simulink model "gm_uz_mpc_3ph"  (R2021a)
settings: Solver=FixedStepDiscrete  StartTime=0.0  StopTime=2000*t_ADC  RelTol=1e-3
undefined symbols (not defined in the file or in its folder): IB, id_ref, iq_ref, lambda_d, lambda_q, lambda_u, Ld_over_LB, Lq_over_LB, n_rpm, omegaB, p, psi_pm_over_psiB, Rs_over_ZB, t_ADC, t_clock, Ts_times_ZB_over_Ld, Ts_times_ZB_over_Lq, v_dc, VB
libraries: nesl_utility x19, simulink x18, fl_lib x15, ee_lib x7, hdlsllib x2, spsAlphaBetaZerotodq0Lib x1
(part 3 of 3)

== system gm_uz_mpc_3ph/inverter_machine/DC_link ==
  Capacitor : fl_lib/Electrical/Electrical Elements/Capacitor  c=C_dc_link uF  r=1e-6 Ohm  g=0 1/Ohm  i_specify=off  i_priority=None  i=0 A  i_nominal_specify=off  i_nominal_unit=A  i_nominal_value=1  v_specify=off  v_priority=None  v=0 V  v_nominal_specify=off  v_nominal_unit=V  v_nominal_value=1  vc_specify=off  vc_priority=High  vc=0 V  vc_nominal_specify=off  vc_nominal_unit=V  vc_nominal_value=1
  PS-Simulink Converter : nesl_utility/PS-Simulink Converter  PhysicalDomain=network_engine_domain  SubClassName=ps_output  LeftPortType=input  RightPortType=output  PseudoPeriodic=off  Frequencies=[]  Unit=1  AffineConversion=off
      settings: SourceProductBaseCode=PW,SS
  Voltage Sensor : fl_lib/Electrical/Electrical Sensors/Voltage Sensor
  U_dc_link+_in : PMIOPort  Side=Left
  U_dc_link-_in : PMIOPort  Port=2  Side=Left
  U_dc_link+_out : PMIOPort  Port=3  Side=Right
  U_dc_link-_out : PMIOPort  Port=4  Side=Right
  u_dc_link_measured : Outport  VectorParamsAs1DForOutWhenUnconnected=off
  wires:
  PS-Simulink Converter/1 -> u_dc_link_measured/1
  connections:
  Voltage Sensor/RConn1 -- PS-Simulink Converter/LConn1
  Capacitor/RConn1 -- U_dc_link-_out/RConn1 -- Voltage Sensor/RConn2 -- U_dc_link-_in/RConn1
  Capacitor/LConn1 -- U_dc_link+_out/RConn1 -- Voltage Sensor/LConn1 -- U_dc_link+_in/RConn1

== system gm_uz_mpc_3ph/inverter_machine/Power_Source ==
  Controlled Voltage Source : fl_lib/Electrical/Electrical Sources/Controlled Voltage Source
  + : PMIOPort  Side=Right
  - : PMIOPort  Port=2  Side=Right
  ref_voltage : PMIOPort  Port=3  Side=Left
  connections:
  Controlled Voltage Source/RConn1 -- ref_voltage/RConn1
  Controlled Voltage Source/RConn2 -- -/RConn1
  Controlled Voltage Source/LConn1 -- +/RConn1

== matlab function gm_uz_mpc_3ph/pu_voltages_vsd/finite_control_set ==
  settings: fimath=fimath('RoundingMethod', 'Floor','OverflowAction', 'Wrap','ProductMode', 'FullPrecision', 'SumMode', 'FullPrecision')
  data: v_DC_pu input; sin_angle input; pu_ud output; pu_uq output; cos_angle input; index input
function [pu_ud,pu_uq] = voltage_space_vectors(v_DC_pu, sin_angle, cos_angle, index)

fm = fimath();
v_DC_pu = fi(v_DC_pu,1,18,15,fm);
sin_angle = fi(sin_angle,1,27,20,fm);
cos_angle = fi(cos_angle,1,27,20,fm);

% u_d-voltages lookup factors alpha/beta
vd_pu = fi([0,0;
    0.666666666666667,0;
    -0.333333333333334,0.577350269189626;
    0.333333333333333,0.577350269189626;
    -0.333333333333333,-0.577350269189626;
    0.333333333333334,-0.577350269189626;
    -0.666666666666667,0;
    0,0],1,18,15);

% u_q-voltages lookup factors alpha/beta
vq_pu = fi([0,0;
    0.666666666666667,0;
    -0.333333333333334,0.577350269189626;
    0.333333333333333,0.577350269189626;
    -0.333333333333333,-0.577350269189626;
    0.333333333333334,-0.577350269189626;
    -0.666666666666667,0;
    0,0],1,18,15);

pu_ud = fi(v_DC_pu * (vd_pu(index,1) * cos_angle + vd_pu(index,2) * sin_angle),1,27,24);
pu_uq = fi(v_DC_pu * (vq_pu(index,1) * -sin_angle + vq_pu(index,2) * cos_angle),1,27,24);

== matlab function gm_uz_mpc_3ph/uz_clarke/clarke ==
  settings: fimath=fimath('RoundingMethod', 'Floor','OverflowAction', 'Wrap','ProductMode', 'FullPrecision', 'SumMode', 'FullPrecision')
  data: a1 input; alpha output; b1 input; c1 input; beta output; zero output
function [alpha,beta,zero] = fcn(a1,b1,c1)


A = [fi(0,1,18,11) fi(0,1,18,11) fi(0,1,18,11)]';

A =    2/3*[1    -0.5        -0.5       ;
           0    sqrt(3)/2   -sqrt(3)/2  ;
           0.5    0.5        0.5] * [a1 b1 c1 ]';

alpha = fi(A(1),1,18,11);
beta = fi(A(2),1,18,11);
zero = fi(A(3),1,18,11);

== matlab function gm_uz_mpc_3ph/cost_opt/MATLAB Function ==
  settings: fimath=fimath('RoundingMethod', 'Floor','OverflowAction', 'Wrap','ProductMode', 'FullPrecision', 'SumMode', 'FullPrecision')
  data: in input; G_next output; index input; last_optim_index input; G_prev output
function [G_next,G_prev] = get_switch_positions(in,index,last_optim_index)
%#codegen
G_next = in(index,[1 3 5]);
G_prev = in(last_optim_index,[1 3 5]);

== matlab function gm_uz_mpc_3ph/cost_opt/iterativesearch ==
  settings: fimath=fimath('RoundingMethod', 'Floor','OverflowAction', 'Wrap','ProductMode', 'FullPrecision', 'SumMode', 'FullPrecision')
  data: index input; opt_idx output; cost input; min_costs output; opt_done output
function [opt_idx,min_costs,opt_done] = fcn(index, cost)
%#codegen

persistent cost_old
if isempty(cost_old)
    cost_old = fi(4.98,0,27,24);
end

persistent index_old
if isempty(index_old)
    index_old = uint32(1);
end

persistent opt_idx_old
if isempty(opt_idx_old)
    opt_idx_old = uint32(1);
end

opt_done = false;

if (index ~= index_old)
    if (index <= 8)
        if (cost <= cost_old)
            opt_idx_old = index; 
            cost_old = cost;
        else
           % do nothing 
        end
    else
   
    end
    
    if (index == 8)
        opt_done = true;
        cost_old = fi(4.98,0,27,24);
    end
    index_old = index;
else
    % do nothing
end

min_costs = cost_old;
opt_idx = opt_idx_old;

== matlab function gm_uz_mpc_3ph/clarke ==
  settings: fimath=fimath('RoundingMethod', 'Floor','OverflowAction', 'Wrap','ProductMode', 'FullPrecision', 'SumMode', 'FullPrecision')
  data: a1 input; alpha output; b1 input; c1 input; beta output; zero output
function [alpha,beta,zero] = fcn(a1,b1,c1)


A = [0 0 0]';

A =    2/3*[1    -0.5        -0.5       ;
           0    sqrt(3)/2   -sqrt(3)/2  ;
           0.5    0.5        0.5] * [a1 b1 c1 ]';

alpha = A(1);
beta = A(2);
zero = A(3);

== matlab function gm_uz_mpc_3ph/cost_opt/FiniteControlSetSwitchingTable ==
  settings: fimath=fimath('RoundingMethod', 'Floor','OverflowAction', 'Wrap','ProductMode', 'FullPrecision', 'SumMode', 'FullPrecision')
  data: G output
function G  = switchingTable

% -------------------------------------------------------------------
%  Generated by MATLAB on 14-Oct-2020 14:52:37
%  MATLAB version: 9.4.0.813654 (R2018a)
% -------------------------------------------------------------------
                                         

s1_v = boolean([0; 1; 0; 1; 0; 1; 0; 1]);


s2_v = boolean([1; 0; 1; 0; 1; 0; 1; 0]);


s3_v = boolean([0; 0; 1; 1; 0; 0; 1; 1]);


s4_v = boolean([1; 1; 0; 0; 1; 1; 0; 0]);


s5_v = boolean([0; 0; 0; 0; 1; 1; 1; 1]);


s6_v = boolean([1; 1; 1; 1; 0; 0; 0; 0]);
     
G = [s1_v, s2_v, s3_v, s4_v, s5_v, s6_v];

== matlab function gm_uz_mpc_3ph/counter_f_sw_3ph/Count_f_sw/Count_f_sw ==
  settings: fimath=fimath('RoundingMethod', 'Floor','OverflowAction', 'Wrap','ProductMode', 'FullPrecision', 'SumMode', 'FullPrecision')
  data: switchNumb input fixdt(0,25,0); ss_v_old input; ss_v input; switchNumbOut output fixdt(0,25,0); bReset input
 function switchNumbOut   = Count_f_sw(switchNumb,ss_v_old,ss_v, bReset)
   %
    %% toDO
        %s
 
    %% Initialization
    Fq25    = fimath('RoundingMethod', 'Floor', 'OverflowAction', 'Wrap','ProductMode', 'FullPrecision', 'ProductWordLength', 25,'ProductFractionLength',0,'SumMode','SpecifyPrecision','SumWordLength',25,'SumFractionLength',0);

    % I need this initialization, in order that the HDL Coder and Simulink knows the size of the vectors! Without these, i will get an error!
   % idx_globalOld     = fi(1, 0, 8, 0); % Chosen position overall in the error vector
    %switchNumb = fi(0, 0, 25, 0);
    
    %% Reset the counters (similar to the THD, i will try to average the switching frequency over 20 fundamental periods. After this time, a Reset-Flag from the ARM processor will reset the counter) 
    if (bReset == true) 
        switchNumb = fi(0, 0, 25, 0);
    end
    %% Check if switching occurs. If yes count up.
    % However, dependent of the ss_v before, switching can but do not have to occure, if the previously applied ss_v keeps.

    %Use a for-loop since in VHDL i have time and can do a resource streaming
    %Even if i need 6 cycles @100MHz, since it is not able to have have
    %switching (on/off inside of 60ns), this is ok (because T_cf = 10us and
    %and switching for such a short time is not allwoed nayway, since it is
    %not worth it (too much losses).)
    for countSS=fi(1, 0, 8, 0):fi(6, 0, 8, 0) %1:6
        if (ss_v(countSS) ~= ss_v_old(countSS)) %Check if switch has changed
            switchNumb = fi(add(Fq25,switchNumb,fi(1, 0, 25, 0)),0,25,0); % +1 Increment the switch counter +1
        end
    end

    switchNumbOut = switchNumb;

 end
